simulink model "gm_uz_pmsm_model_9ph_21b_all_double_vnl"  (R2021b)
settings: Solver=FixedStepDiscrete  StartTime=0.0  StopTime=0.8  RelTol=1e-3
PreLoadFcn:
  | uz_pmsm_model_9ph_init_parameter
undefined symbols (not defined in the file or in its folder): a, b, c, friction_coefficient, inertia, k_i_d, k_i_q, k_p_d, k_p_q, Kpd, L_d, L_o1, L_o2, L_q, L_x1, L_x2, L_y1, L_y2, L_zero, polepair, psi_pm, R_1, static_friction_torque, Tnd, ts
libraries: hdlmdlgenlib x139, hdlsllib x90, dspsigops x21, simulink x17, slpidlib x2, spsAlphaBetaZerotodq0Lib x1, pid_lib x1, spsdq0toAlphaBetaZeroLib x1
(part 5 of 5)

== system gm_uz_pmsm_model_9ph_21b_all_double_vnl/uz_pmsm_model_9ph/dq_model_9ph/Data Type Conversion7 ==
  In1 : Inport
  Data Type Conversion7 : DataTypeConversion  OutDataTypeStr=double  RndMeth=Nearest  SampleTime=1e-08
  Data Type Conversion7_pd1 : Delay  DelayLength=3
  Out1 : Outport
  wires:
  Data Type Conversion7_pd1/1 -> Out1/1
  Data Type Conversion7/1 -> Data Type Conversion7_pd1/1
  In1/1 -> Data Type Conversion7/1

== system gm_uz_pmsm_model_9ph_21b_all_double_vnl/uz_pmsm_model_9ph/dq_model_9ph/Data Type Conversion71 ==
  In1 : Inport
  Data Type Conversion71 : DataTypeConversion  OutDataTypeStr=double  RndMeth=Nearest  SampleTime=1e-08
  Data Type Conversion71_pd1 : Delay  DelayLength=3
  Out1 : Outport
  wires:
  Data Type Conversion71_pd1/1 -> Out1/1
  Data Type Conversion71/1 -> Data Type Conversion71_pd1/1
  In1/1 -> Data Type Conversion71/1

== system gm_uz_pmsm_model_9ph_21b_all_double_vnl/uz_pmsm_model_9ph/dq_model_9ph/Data Type Conversion8 ==
  In1 : Inport
  Data Type Conversion8 : DataTypeConversion  OutDataTypeStr=double  RndMeth=Nearest  SampleTime=1e-08
  Data Type Conversion8_pd1 : Delay  DelayLength=3
  Out1 : Outport
  wires:
  Data Type Conversion8_pd1/1 -> Out1/1
  Data Type Conversion8/1 -> Data Type Conversion8_pd1/1
  In1/1 -> Data Type Conversion8/1

== system gm_uz_pmsm_model_9ph_21b_all_double_vnl/uz_pmsm_model_9ph/dq_model_9ph/Data Type Conversion9 ==
  In1 : Inport
  Data Type Conversion9 : DataTypeConversion  OutDataTypeStr=double  RndMeth=Nearest  SampleTime=1e-08
  Data Type Conversion9_pd1 : Delay  DelayLength=3
  Out1 : Outport
  wires:
  Data Type Conversion9_pd1/1 -> Out1/1
  Data Type Conversion9/1 -> Data Type Conversion9_pd1/1
  In1/1 -> Data Type Conversion9/1

== system gm_uz_pmsm_model_9ph_21b_all_double_vnl/uz_pmsm_model_9ph/dq_model_9ph/Divide ==
  In1 : Inport
  In2 : Inport  Port=2
  Divide : Product  Inputs=**  OutDataTypeStr=double  SampleTime=1e-08
  Divide_pd1 : Delay  DelayLength=6
  Out1 : Outport
  wires:
  Divide_pd1/1 -> Out1/1
  Divide/1 -> Divide_pd1/1
  In2/1 -> Divide/2
  In1/1 -> Divide/1

== system gm_uz_pmsm_model_9ph_21b_all_double_vnl/uz_pmsm_model_9ph/dq_model_9ph/Divide1 ==
  In1 : Inport
  In2 : Inport  Port=2
  Divide1 : Product  Inputs=**  OutDataTypeStr=double  SampleTime=1e-08
  Divide1_pd1 : Delay  DelayLength=6
  Out1 : Outport
  wires:
  Divide1_pd1/1 -> Out1/1
  Divide1/1 -> Divide1_pd1/1
  In2/1 -> Divide1/2
  In1/1 -> Divide1/1

== system gm_uz_pmsm_model_9ph_21b_all_double_vnl/uz_pmsm_model_9ph/dq_model_9ph/Divide10 ==
  In1 : Inport
  In2 : Inport  Port=2
  Divide10 : Product  Inputs=**  OutDataTypeStr=double  SampleTime=1e-08
  Divide10_pd1 : Delay  DelayLength=6
  Out1 : Outport
  wires:
  Divide10_pd1/1 -> Out1/1
  Divide10/1 -> Divide10_pd1/1
  In2/1 -> Divide10/2
  In1/1 -> Divide10/1

== system gm_uz_pmsm_model_9ph_21b_all_double_vnl/uz_pmsm_model_9ph/dq_model_9ph/Divide11 ==
  In1 : Inport
  In2 : Inport  Port=2
  Divide11 : Product  Inputs=**  OutDataTypeStr=double  SampleTime=1e-08
  Divide11_pd1 : Delay  DelayLength=6
  Out1 : Outport
  wires:
  Divide11_pd1/1 -> Out1/1
  Divide11/1 -> Divide11_pd1/1
  In2/1 -> Divide11/2
  In1/1 -> Divide11/1

== system gm_uz_pmsm_model_9ph_21b_all_double_vnl/uz_pmsm_model_9ph/dq_model_9ph/Divide12 ==
  In1 : Inport
  In2 : Inport  Port=2
  Divide12 : Product  Inputs=**  OutDataTypeStr=double  SampleTime=1e-08
  Divide12_pd1 : Delay  DelayLength=6
  Out1 : Outport
  wires:
  Divide12_pd1/1 -> Out1/1
  Divide12/1 -> Divide12_pd1/1
  In2/1 -> Divide12/2
  In1/1 -> Divide12/1

== system gm_uz_pmsm_model_9ph_21b_all_double_vnl/uz_pmsm_model_9ph/dq_model_9ph/Divide13 ==
  In1 : Inport
  In2 : Inport  Port=2
  Divide13 : Product  Inputs=**  OutDataTypeStr=double  SampleTime=1e-08
  Divide13_pd1 : Delay  DelayLength=6
  Out1 : Outport
  wires:
  Divide13_pd1/1 -> Out1/1
  Divide13/1 -> Divide13_pd1/1
  In2/1 -> Divide13/2
  In1/1 -> Divide13/1

== system gm_uz_pmsm_model_9ph_21b_all_double_vnl/uz_pmsm_model_9ph/dq_model_9ph/Divide2 ==
  In1 : Inport
  In2 : Inport  Port=2
  Divide2 : Product  Inputs=**  OutDataTypeStr=double  SampleTime=1e-08
  Divide2_pd1 : Delay  DelayLength=6
  Out1 : Outport
  wires:
  Divide2_pd1/1 -> Out1/1
  Divide2/1 -> Divide2_pd1/1
  In2/1 -> Divide2/2
  In1/1 -> Divide2/1

== system gm_uz_pmsm_model_9ph_21b_all_double_vnl/uz_pmsm_model_9ph/dq_model_9ph/Divide3 ==
  In1 : Inport
  In2 : Inport  Port=2
  Divide3 : Product  Inputs=**  OutDataTypeStr=double  SampleTime=1e-08
  Divide3_pd1 : Delay  DelayLength=6
  Out1 : Outport
  wires:
  Divide3_pd1/1 -> Out1/1
  Divide3/1 -> Divide3_pd1/1
  In2/1 -> Divide3/2
  In1/1 -> Divide3/1

== system gm_uz_pmsm_model_9ph_21b_all_double_vnl/uz_pmsm_model_9ph/dq_model_9ph/Divide4 ==
  In1 : Inport
  In2 : Inport  Port=2
  Divide4 : Product  Inputs=**  OutDataTypeStr=double  SampleTime=1e-08
  Divide4_pd1 : Delay  DelayLength=6
  Out1 : Outport
  wires:
  Divide4_pd1/1 -> Out1/1
  Divide4/1 -> Divide4_pd1/1
  In2/1 -> Divide4/2
  In1/1 -> Divide4/1

== system gm_uz_pmsm_model_9ph_21b_all_double_vnl/uz_pmsm_model_9ph/dq_model_9ph/Divide5 ==
  In1 : Inport
  In2 : Inport  Port=2
  Divide5 : Product  Inputs=**  OutDataTypeStr=double  SampleTime=1e-08
  Divide5_pd1 : Delay  DelayLength=6
  Out1 : Outport
  wires:
  Divide5_pd1/1 -> Out1/1
  Divide5/1 -> Divide5_pd1/1
  In2/1 -> Divide5/2
  In1/1 -> Divide5/1

== system gm_uz_pmsm_model_9ph_21b_all_double_vnl/uz_pmsm_model_9ph/dq_model_9ph/Divide6 ==
  In1 : Inport
  In2 : Inport  Port=2
  Divide6 : Product  Inputs=**  OutDataTypeStr=double  SampleTime=1e-08
  Divide6_pd1 : Delay  DelayLength=6
  Out1 : Outport
  wires:
  Divide6_pd1/1 -> Out1/1
  Divide6/1 -> Divide6_pd1/1
  In2/1 -> Divide6/2
  In1/1 -> Divide6/1

== system gm_uz_pmsm_model_9ph_21b_all_double_vnl/uz_pmsm_model_9ph/dq_model_9ph/Divide7 ==
  In1 : Inport
  In2 : Inport  Port=2
  Divide7 : Product  Inputs=**  OutDataTypeStr=double  SampleTime=1e-08
  Divide7_pd1 : Delay  DelayLength=6
  Out1 : Outport
  wires:
  Divide7_pd1/1 -> Out1/1
  Divide7/1 -> Divide7_pd1/1
  In2/1 -> Divide7/2
  In1/1 -> Divide7/1

== system gm_uz_pmsm_model_9ph_21b_all_double_vnl/uz_pmsm_model_9ph/dq_model_9ph/Divide8 ==
  In1 : Inport
  In2 : Inport  Port=2
  Divide8 : Product  Inputs=**  OutDataTypeStr=double  SampleTime=1e-08
  Divide8_pd1 : Delay  DelayLength=6
  Out1 : Outport
  wires:
  Divide8_pd1/1 -> Out1/1
  Divide8/1 -> Divide8_pd1/1
  In2/1 -> Divide8/2
  In1/1 -> Divide8/1

== system gm_uz_pmsm_model_9ph_21b_all_double_vnl/uz_pmsm_model_9ph/dq_model_9ph/Divide9 ==
  In1 : Inport
  In2 : Inport  Port=2
  Divide9 : Product  Inputs=**  OutDataTypeStr=double  SampleTime=1e-08
  Divide9_pd1 : Delay  DelayLength=6
  Out1 : Outport
  wires:
  Divide9_pd1/1 -> Out1/1
  Divide9/1 -> Divide9_pd1/1
  In2/1 -> Divide9/2
  In1/1 -> Divide9/1

== system gm_uz_pmsm_model_9ph_21b_all_double_vnl/uz_pmsm_model_9ph/dq_model_9ph/Factor ==
  In1 : Inport
  In2 : Inport  Port=2
  Factor : Product  Inputs=**  OutDataTypeStr=double  SampleTime=1e-08
  Factor_pd1 : Delay  DelayLength=6
  Out1 : Outport
  wires:
  Factor_pd1/1 -> Out1/1
  Factor/1 -> Factor_pd1/1
  In2/1 -> Factor/2
  In1/1 -> Factor/1

== system gm_uz_pmsm_model_9ph_21b_all_double_vnl/uz_pmsm_model_9ph/dq_model_9ph/Gain ==
  In1 : Inport
  In2 : Inport  Port=2
  Gain : Product  Inputs=**  OutDataTypeStr=double  SampleTime=1e-08
  Gain_pd1 : Delay  DelayLength=6
  Out1 : Outport
  wires:
  Gain_pd1/1 -> Out1/1
  Gain/1 -> Gain_pd1/1
  In2/1 -> Gain/2
  In1/1 -> Gain/1

== system gm_uz_pmsm_model_9ph_21b_all_double_vnl/uz_pmsm_model_9ph/dq_model_9ph/Gain1 ==
  In1 : Inport
  In2 : Inport  Port=2
  Gain1 : Product  Inputs=**  OutDataTypeStr=double  SampleTime=1e-08
  Gain1_pd1 : Delay  DelayLength=6
  Out1 : Outport
  wires:
  Gain1_pd1/1 -> Out1/1
  Gain1/1 -> Gain1_pd1/1
  In2/1 -> Gain1/2
  In1/1 -> Gain1/1

== system gm_uz_pmsm_model_9ph_21b_all_double_vnl/uz_pmsm_model_9ph/dq_model_9ph/Gain10 ==
  In1 : Inport
  In2 : Inport  Port=2
  Gain10 : Product  Inputs=**  OutDataTypeStr=double  SampleTime=1e-08
  Gain10_pd1 : Delay  DelayLength=6
  Out1 : Outport
  wires:
  Gain10_pd1/1 -> Out1/1
  Gain10/1 -> Gain10_pd1/1
  In2/1 -> Gain10/2
  In1/1 -> Gain10/1

== system gm_uz_pmsm_model_9ph_21b_all_double_vnl/uz_pmsm_model_9ph/dq_model_9ph/Gain2 ==
  In1 : Inport
  In2 : Inport  Port=2
  Gain2 : Product  Inputs=**  OutDataTypeStr=double  SampleTime=1e-08
  Gain2_pd1 : Delay  DelayLength=6
  Out1 : Outport
  wires:
  Gain2_pd1/1 -> Out1/1
  Gain2/1 -> Gain2_pd1/1
  In2/1 -> Gain2/2
  In1/1 -> Gain2/1

== system gm_uz_pmsm_model_9ph_21b_all_double_vnl/uz_pmsm_model_9ph/dq_model_9ph/Gain3 ==
  In1 : Inport
  In2 : Inport  Port=2
  Gain3 : Product  Inputs=**  OutDataTypeStr=double  SampleTime=1e-08
  Gain3_pd1 : Delay  DelayLength=6
  Out1 : Outport
  wires:
  Gain3_pd1/1 -> Out1/1
  Gain3/1 -> Gain3_pd1/1
  In2/1 -> Gain3/2
  In1/1 -> Gain3/1

== system gm_uz_pmsm_model_9ph_21b_all_double_vnl/uz_pmsm_model_9ph/dq_model_9ph/Gain4 ==
  In1 : Inport
  In2 : Inport  Port=2
  Gain4 : Product  Inputs=**  OutDataTypeStr=double  SampleTime=1e-08
  Gain4_pd1 : Delay  DelayLength=6
  Out1 : Outport
  wires:
  Gain4_pd1/1 -> Out1/1
  Gain4/1 -> Gain4_pd1/1
  In2/1 -> Gain4/2
  In1/1 -> Gain4/1

== system gm_uz_pmsm_model_9ph_21b_all_double_vnl/uz_pmsm_model_9ph/dq_model_9ph/Gain5 ==
  In1 : Inport
  In2 : Inport  Port=2
  Gain5 : Product  Inputs=**  OutDataTypeStr=double  SampleTime=1e-08
  Gain5_pd1 : Delay  DelayLength=6
  Out1 : Outport
  wires:
  Gain5_pd1/1 -> Out1/1
  Gain5/1 -> Gain5_pd1/1
  In2/1 -> Gain5/2
  In1/1 -> Gain5/1

== system gm_uz_pmsm_model_9ph_21b_all_double_vnl/uz_pmsm_model_9ph/dq_model_9ph/Gain6 ==
  In1 : Inport
  In2 : Inport  Port=2
  Gain6 : Product  Inputs=**  OutDataTypeStr=double  SampleTime=1e-08
  Gain6_pd1 : Delay  DelayLength=6
  Out1 : Outport
  wires:
  Gain6_pd1/1 -> Out1/1
  Gain6/1 -> Gain6_pd1/1
  In2/1 -> Gain6/2
  In1/1 -> Gain6/1

== system gm_uz_pmsm_model_9ph_21b_all_double_vnl/uz_pmsm_model_9ph/dq_model_9ph/Gain7 ==
  In1 : Inport
  In2 : Inport  Port=2
  Gain7 : Product  Inputs=**  OutDataTypeStr=double  SampleTime=1e-08
  Gain7_pd1 : Delay  DelayLength=6
  Out1 : Outport
  wires:
  Gain7_pd1/1 -> Out1/1
  Gain7/1 -> Gain7_pd1/1
  In2/1 -> Gain7/2
  In1/1 -> Gain7/1

== system gm_uz_pmsm_model_9ph_21b_all_double_vnl/uz_pmsm_model_9ph/dq_model_9ph/Gain8 ==
  In1 : Inport
  In2 : Inport  Port=2
  Gain8 : Product  Inputs=**  OutDataTypeStr=double  SampleTime=1e-08
  Gain8_pd1 : Delay  DelayLength=6
  Out1 : Outport
  wires:
  Gain8_pd1/1 -> Out1/1
  Gain8/1 -> Gain8_pd1/1
  In2/1 -> Gain8/2
  In1/1 -> Gain8/1

== system gm_uz_pmsm_model_9ph_21b_all_double_vnl/uz_pmsm_model_9ph/dq_model_9ph/Gain9 ==
  In1 : Inport
  In2 : Inport  Port=2
  Gain9 : Product  Inputs=**  OutDataTypeStr=double  SampleTime=1e-08
  Gain9_pd1 : Delay  DelayLength=6
  Out1 : Outport
  wires:
  Gain9_pd1/1 -> Out1/1
  Gain9/1 -> Gain9_pd1/1
  In2/1 -> Gain9/2
  In1/1 -> Gain9/1

== system gm_uz_pmsm_model_9ph_21b_all_double_vnl/uz_pmsm_model_9ph/dq_model_9ph/Product ==
  In1 : Inport
  In2 : Inport  Port=2
  Product : Product  Inputs=**  OutDataTypeStr=double  SampleTime=1e-08
  Product_pd1 : Delay  DelayLength=6
  Out1 : Outport
  wires:
  Product_pd1/1 -> Out1/1
  Product/1 -> Product_pd1/1
  In2/1 -> Product/2
  In1/1 -> Product/1

== system gm_uz_pmsm_model_9ph_21b_all_double_vnl/uz_pmsm_model_9ph/dq_model_9ph/Product1 ==
  In1 : Inport
  In2 : Inport  Port=2
  Product1 : Product  Inputs=**  OutDataTypeStr=double  SampleTime=1e-08
  Product1_pd1 : Delay  DelayLength=6
  Out1 : Outport
  wires:
  Product1_pd1/1 -> Out1/1
  Product1/1 -> Product1_pd1/1
  In2/1 -> Product1/2
  In1/1 -> Product1/1

== system gm_uz_pmsm_model_9ph_21b_all_double_vnl/uz_pmsm_model_9ph/dq_model_9ph/Product10 ==
  In1 : Inport
  In2 : Inport  Port=2
  Product10 : Product  Inputs=**  OutDataTypeStr=double  SampleTime=1e-08
  Product10_pd1 : Delay  DelayLength=6
  Out1 : Outport
  wires:
  Product10_pd1/1 -> Out1/1
  Product10/1 -> Product10_pd1/1
  In2/1 -> Product10/2
  In1/1 -> Product10/1

== system gm_uz_pmsm_model_9ph_21b_all_double_vnl/uz_pmsm_model_9ph/dq_model_9ph/Product11 ==
  In1 : Inport
  In2 : Inport  Port=2
  Product11 : Product  Inputs=**  OutDataTypeStr=double  SampleTime=1e-08
  Product11_pd1 : Delay  DelayLength=6
  Out1 : Outport
  wires:
  Product11_pd1/1 -> Out1/1
  Product11/1 -> Product11_pd1/1
  In2/1 -> Product11/2
  In1/1 -> Product11/1

== system gm_uz_pmsm_model_9ph_21b_all_double_vnl/uz_pmsm_model_9ph/dq_model_9ph/Product2 ==
  In1 : Inport
  In2 : Inport  Port=2
  Product2 : Product  Inputs=**  OutDataTypeStr=double  SampleTime=1e-08
  Product2_pd1 : Delay  DelayLength=6
  Out1 : Outport
  wires:
  Product2_pd1/1 -> Out1/1
  Product2/1 -> Product2_pd1/1
  In2/1 -> Product2/2
  In1/1 -> Product2/1

== system gm_uz_pmsm_model_9ph_21b_all_double_vnl/uz_pmsm_model_9ph/dq_model_9ph/Product3 ==
  In1 : Inport
  In2 : Inport  Port=2
  Product3 : Product  Inputs=**  OutDataTypeStr=double  SampleTime=1e-08
  Product3_pd1 : Delay  DelayLength=6
  Out1 : Outport
  wires:
  Product3_pd1/1 -> Out1/1
  Product3/1 -> Product3_pd1/1
  In2/1 -> Product3/2
  In1/1 -> Product3/1

== system gm_uz_pmsm_model_9ph_21b_all_double_vnl/uz_pmsm_model_9ph/dq_model_9ph/Product4 ==
  In1 : Inport
  In2 : Inport  Port=2
  Product4 : Product  Inputs=**  OutDataTypeStr=double  SampleTime=1e-08
  Product4_pd1 : Delay  DelayLength=6
  Out1 : Outport
  wires:
  Product4_pd1/1 -> Out1/1
  Product4/1 -> Product4_pd1/1
  In2/1 -> Product4/2
  In1/1 -> Product4/1

== system gm_uz_pmsm_model_9ph_21b_all_double_vnl/uz_pmsm_model_9ph/dq_model_9ph/Product5 ==
  In1 : Inport
  In2 : Inport  Port=2
  Product5 : Product  Inputs=**  OutDataTypeStr=double  SampleTime=1e-08
  Product5_pd1 : Delay  DelayLength=6
  Out1 : Outport
  wires:
  Product5_pd1/1 -> Out1/1
  Product5/1 -> Product5_pd1/1
  In2/1 -> Product5/2
  In1/1 -> Product5/1

== system gm_uz_pmsm_model_9ph_21b_all_double_vnl/uz_pmsm_model_9ph/dq_model_9ph/Product6 ==
  In1 : Inport
  In2 : Inport  Port=2
  Product6 : Product  Inputs=**  OutDataTypeStr=double  SampleTime=1e-08
  Product6_pd1 : Delay  DelayLength=6
  Out1 : Outport
  wires:
  Product6_pd1/1 -> Out1/1
  Product6/1 -> Product6_pd1/1
  In2/1 -> Product6/2
  In1/1 -> Product6/1

== system gm_uz_pmsm_model_9ph_21b_all_double_vnl/uz_pmsm_model_9ph/dq_model_9ph/Product7 ==
  In1 : Inport
  In2 : Inport  Port=2
  Product7 : Product  Inputs=**  OutDataTypeStr=double  SampleTime=1e-08
  Product7_pd1 : Delay  DelayLength=6
  Out1 : Outport
  wires:
  Product7_pd1/1 -> Out1/1
  Product7/1 -> Product7_pd1/1
  In2/1 -> Product7/2
  In1/1 -> Product7/1

== system gm_uz_pmsm_model_9ph_21b_all_double_vnl/uz_pmsm_model_9ph/dq_model_9ph/Product8 ==
  In1 : Inport
  In2 : Inport  Port=2
  Product8 : Product  Inputs=**  OutDataTypeStr=double  SampleTime=1e-08
  Product8_pd1 : Delay  DelayLength=6
  Out1 : Outport
  wires:
  Product8_pd1/1 -> Out1/1
  Product8/1 -> Product8_pd1/1
  In2/1 -> Product8/2
  In1/1 -> Product8/1

== system gm_uz_pmsm_model_9ph_21b_all_double_vnl/uz_pmsm_model_9ph/dq_model_9ph/Product9 ==
  In1 : Inport
  In2 : Inport  Port=2
  Product9 : Product  Inputs=**  OutDataTypeStr=double  SampleTime=1e-08
  Product9_pd1 : Delay  DelayLength=6
  Out1 : Outport
  wires:
  Product9_pd1/1 -> Out1/1
  Product9/1 -> Product9_pd1/1
  In2/1 -> Product9/2
  In1/1 -> Product9/1

== system gm_uz_pmsm_model_9ph_21b_all_double_vnl/uz_pmsm_model_9ph/dq_model_9ph/Sum ==
  In1 : Inport
  In2 : Inport  Port=2
  Sum : Sum  OutDataTypeStr=double  SampleTime=1e-08
  Sum_pd1 : Delay  DelayLength=6
  Out1 : Outport
  wires:
  Sum_pd1/1 -> Out1/1
  Sum/1 -> Sum_pd1/1
  In2/1 -> Sum/2
  In1/1 -> Sum/1

== system gm_uz_pmsm_model_9ph_21b_all_double_vnl/uz_pmsm_model_9ph/dq_model_9ph/Sum1 ==
  In1 : Inport
  In2 : Inport  Port=2
  Sum1 : Sum  Inputs=+-  OutDataTypeStr=double  SampleTime=1e-08
  Sum1_pd1 : Delay  DelayLength=6
  Out1 : Outport
  wires:
  Sum1_pd1/1 -> Out1/1
  Sum1/1 -> Sum1_pd1/1
  In2/1 -> Sum1/2
  In1/1 -> Sum1/1

== system gm_uz_pmsm_model_9ph_21b_all_double_vnl/uz_pmsm_model_9ph/dq_model_9ph/Sum11 ==
  In1 : Inport
  In2 : Inport  Port=2
  Sum11 : Sum  OutDataTypeStr=double  SampleTime=1e-08
  Sum11_pd1 : Delay  DelayLength=6
  Out1 : Outport
  wires:
  Sum11_pd1/1 -> Out1/1
  Sum11/1 -> Sum11_pd1/1
  In2/1 -> Sum11/2
  In1/1 -> Sum11/1

== system gm_uz_pmsm_model_9ph_21b_all_double_vnl/uz_pmsm_model_9ph/dq_model_9ph/Sum1_stage2 ==
  In1 : Inport
  In2 : Inport  Port=2
  Sum1_stage2 : Sum  Inputs=+-  OutDataTypeStr=double  SampleTime=1e-08
  Sum1_stage2_pd1 : Delay  DelayLength=6
  Out1 : Outport
  wires:
  Sum1_stage2_pd1/1 -> Out1/1
  Sum1_stage2/1 -> Sum1_stage2_pd1/1
  In2/1 -> Sum1_stage2/2
  In1/1 -> Sum1_stage2/1

== system gm_uz_pmsm_model_9ph_21b_all_double_vnl/uz_pmsm_model_9ph/dq_model_9ph/Sum1_stage3 ==
  In1 : Inport
  In2 : Inport  Port=2
  Sum1_stage3 : Sum  Inputs=+-  OutDataTypeStr=double  SampleTime=1e-08
  Sum1_stage3_pd1 : Delay  DelayLength=6
  Out1 : Outport
  wires:
  Sum1_stage3_pd1/1 -> Out1/1
  Sum1_stage3/1 -> Sum1_stage3_pd1/1
  In2/1 -> Sum1_stage3/2
  In1/1 -> Sum1_stage3/1

== system gm_uz_pmsm_model_9ph_21b_all_double_vnl/uz_pmsm_model_9ph/dq_model_9ph/Sum2 ==
  In1 : Inport
  In2 : Inport  Port=2
  Sum2 : Sum  OutDataTypeStr=double  SampleTime=1e-08
  Sum2_pd1 : Delay  DelayLength=6
  Out1 : Outport
  wires:
  Sum2_pd1/1 -> Out1/1
  Sum2/1 -> Sum2_pd1/1
  In2/1 -> Sum2/2
  In1/1 -> Sum2/1

== system gm_uz_pmsm_model_9ph_21b_all_double_vnl/uz_pmsm_model_9ph/dq_model_9ph/Sum21 ==
  In1 : Inport
  In2 : Inport  Port=2
  Sum21 : Sum  Inputs=+-  OutDataTypeStr=double  SampleTime=1e-08
  Sum21_pd1 : Delay  DelayLength=6
  Out1 : Outport
  wires:
  Sum21_pd1/1 -> Out1/1
  Sum21/1 -> Sum21_pd1/1
  In2/1 -> Sum21/2
  In1/1 -> Sum21/1

== system gm_uz_pmsm_model_9ph_21b_all_double_vnl/uz_pmsm_model_9ph/dq_model_9ph/Sum3 ==
  In1 : Inport
  In2 : Inport  Port=2
  Sum3 : Sum  OutDataTypeStr=double  SampleTime=1e-08
  Sum3_pd1 : Delay  DelayLength=6
  Out1 : Outport
  wires:
  Sum3_pd1/1 -> Out1/1
  Sum3/1 -> Sum3_pd1/1
  In2/1 -> Sum3/2
  In1/1 -> Sum3/1

== system gm_uz_pmsm_model_9ph_21b_all_double_vnl/uz_pmsm_model_9ph/dq_model_9ph/Sum31 ==
  In1 : Inport
  In2 : Inport  Port=2
  Sum31 : Sum  OutDataTypeStr=double  SampleTime=1e-08
  Sum31_pd1 : Delay  DelayLength=6
  Out1 : Outport
  wires:
  Sum31_pd1/1 -> Out1/1
  Sum31/1 -> Sum31_pd1/1
  In2/1 -> Sum31/2
  In1/1 -> Sum31/1

== system gm_uz_pmsm_model_9ph_21b_all_double_vnl/uz_pmsm_model_9ph/dq_model_9ph/Sum310 ==
  In1 : Inport
  In2 : Inport  Port=2
  Sum310 : Sum  OutDataTypeStr=double  SampleTime=1e-08
  Sum310_pd1 : Delay  DelayLength=6
  Out1 : Outport
  wires:
  Sum310_pd1/1 -> Out1/1
  Sum310/1 -> Sum310_pd1/1
  In2/1 -> Sum310/2
  In1/1 -> Sum310/1

== system gm_uz_pmsm_model_9ph_21b_all_double_vnl/uz_pmsm_model_9ph/dq_model_9ph/Sum32 ==
  In1 : Inport
  In2 : Inport  Port=2
  Sum32 : Sum  OutDataTypeStr=double  SampleTime=1e-08
  Sum32_pd1 : Delay  DelayLength=6
  Out1 : Outport
  wires:
  Sum32_pd1/1 -> Out1/1
  Sum32/1 -> Sum32_pd1/1
  In2/1 -> Sum32/2
  In1/1 -> Sum32/1

== system gm_uz_pmsm_model_9ph_21b_all_double_vnl/uz_pmsm_model_9ph/dq_model_9ph/Sum33 ==
  In1 : Inport
  In2 : Inport  Port=2
  Sum33 : Sum  OutDataTypeStr=double  SampleTime=1e-08
  Sum33_pd1 : Delay  DelayLength=6
  Out1 : Outport
  wires:
  Sum33_pd1/1 -> Out1/1
  Sum33/1 -> Sum33_pd1/1
  In2/1 -> Sum33/2
  In1/1 -> Sum33/1

== system gm_uz_pmsm_model_9ph_21b_all_double_vnl/uz_pmsm_model_9ph/dq_model_9ph/Sum34 ==
  In1 : Inport
  In2 : Inport  Port=2
  Sum34 : Sum  OutDataTypeStr=double  SampleTime=1e-08
  Sum34_pd1 : Delay  DelayLength=6
  Out1 : Outport
  wires:
  Sum34_pd1/1 -> Out1/1
  Sum34/1 -> Sum34_pd1/1
  In2/1 -> Sum34/2
  In1/1 -> Sum34/1

== system gm_uz_pmsm_model_9ph_21b_all_double_vnl/uz_pmsm_model_9ph/dq_model_9ph/Sum35 ==
  In1 : Inport
  In2 : Inport  Port=2
  Sum35 : Sum  OutDataTypeStr=double  SampleTime=1e-08
  Sum35_pd1 : Delay  DelayLength=6
  Out1 : Outport
  wires:
  Sum35_pd1/1 -> Out1/1
  Sum35/1 -> Sum35_pd1/1
  In2/1 -> Sum35/2
  In1/1 -> Sum35/1

== system gm_uz_pmsm_model_9ph_21b_all_double_vnl/uz_pmsm_model_9ph/dq_model_9ph/Sum36 ==
  In1 : Inport
  In2 : Inport  Port=2
  Sum36 : Sum  OutDataTypeStr=double  SampleTime=1e-08
  Sum36_pd1 : Delay  DelayLength=6
  Out1 : Outport
  wires:
  Sum36_pd1/1 -> Out1/1
  Sum36/1 -> Sum36_pd1/1
  In2/1 -> Sum36/2
  In1/1 -> Sum36/1

== system gm_uz_pmsm_model_9ph_21b_all_double_vnl/uz_pmsm_model_9ph/dq_model_9ph/Sum37 ==
  In1 : Inport
  In2 : Inport  Port=2
  Sum37 : Sum  OutDataTypeStr=double  SampleTime=1e-08
  Sum37_pd1 : Delay  DelayLength=6
  Out1 : Outport
  wires:
  Sum37_pd1/1 -> Out1/1
  Sum37/1 -> Sum37_pd1/1
  In2/1 -> Sum37/2
  In1/1 -> Sum37/1

== system gm_uz_pmsm_model_9ph_21b_all_double_vnl/uz_pmsm_model_9ph/dq_model_9ph/Sum38 ==
  In1 : Inport
  In2 : Inport  Port=2
  Sum38 : Sum  Inputs=+-  OutDataTypeStr=double  SampleTime=1e-08
  Sum38_pd1 : Delay  DelayLength=6
  Out1 : Outport
  wires:
  Sum38_pd1/1 -> Out1/1
  Sum38/1 -> Sum38_pd1/1
  In2/1 -> Sum38/2
  In1/1 -> Sum38/1

== system gm_uz_pmsm_model_9ph_21b_all_double_vnl/uz_pmsm_model_9ph/dq_model_9ph/Sum39 ==
  In1 : Inport
  In2 : Inport  Port=2
  Sum39 : Sum  OutDataTypeStr=double  SampleTime=1e-08
  Sum39_pd1 : Delay  DelayLength=6
  Out1 : Outport
  wires:
  Sum39_pd1/1 -> Out1/1
  Sum39/1 -> Sum39_pd1/1
  In2/1 -> Sum39/2
  In1/1 -> Sum39/1

== system gm_uz_pmsm_model_9ph_21b_all_double_vnl/uz_pmsm_model_9ph/dq_model_9ph/Sum_stage2 ==
  In1 : Inport
  In2 : Inport  Port=2
  Sum_stage2 : Sum  Inputs=+-  OutDataTypeStr=double  SampleTime=1e-08
  Sum_stage2_pd1 : Delay  DelayLength=6
  Out1 : Outport
  wires:
  Sum_stage2_pd1/1 -> Out1/1
  Sum_stage2/1 -> Sum_stage2_pd1/1
  In2/1 -> Sum_stage2/2
  In1/1 -> Sum_stage2/1

== system gm_uz_pmsm_model_9ph_21b_all_double_vnl/uz_pmsm_model_9ph/dq_model_9ph/Sum_stage3 ==
  In1 : Inport
  In2 : Inport  Port=2
  Sum_stage3 : Sum  OutDataTypeStr=double  SampleTime=1e-08
  Sum_stage3_pd1 : Delay  DelayLength=6
  Out1 : Outport
  wires:
  Sum_stage3_pd1/1 -> Out1/1
  Sum_stage3/1 -> Sum_stage3_pd1/1
  In2/1 -> Sum_stage3/2
  In1/1 -> Sum_stage3/1

== system gm_uz_pmsm_model_9ph_21b_all_double_vnl/uz_pmsm_model_9ph_vnl/Line-Line to Phase voltage/abc   to   alpha_beta_0 ==
  "a, b, c" : Inport  PortDimensions=3
  Gain2 : Gain  Gain=2/3  ParamDataTypeStr=fixdt(1,18,16)  SaturateOnIntegerOverflow=on  OutDataTypeStr=Inherit: Same as input
  Gain4 : Gain  Gain="[ 1   -0.5   -0.5; 0   0.5*sqrt(3)   -0.5*sqrt(3); 0.5  0.5  0.5 ]"  Multiplication=Matrix(K*u) (u vector)  ParamDataTypeStr=fixdt(1,18,16)  OutDataTypeStr=fixdt(1,25,12)  SaturateOnIntegerOverflow=on
  "alpha, beta, 0 " : Outport
  wires:
  Gain4/1 -> Gain2/1
  "a, b, c"/1 -> Gain4/1
  Gain2/1 -> "alpha, beta, 0 "/1

== system gm_uz_pmsm_model_9ph_21b_all_double_vnl/uz_pmsm_model_9ph_vnl/Line-Line to Phase voltage/alpha_beta_0   to   abc ==
  "alpha, beta, 0  " : Inport  PortDimensions=3
  Gain4 : Gain  Gain="[ 1 0 1; -0.5   0.5*sqrt(3)  1; -0.5 -0.5*sqrt(3) 1 ]"  Multiplication=Matrix(K*u) (u vector)  ParamDataTypeStr=fixdt(1,18,16)  SaturateOnIntegerOverflow=on  OutDataTypeStr=Inherit: Same as input
  "a, b, c" : Outport
  wires:
  "alpha, beta, 0  "/1 -> Gain4/1
  Gain4/1 -> "a, b, c"/1

== system gm_uz_pmsm_model_9ph_21b_all_double_vnl/uz_pmsm_model_9ph_vnl/Line-Line to Phase voltage1/abc   to   alpha_beta_0 ==
  "a, b, c" : Inport  PortDimensions=3
  Gain2 : Gain  Gain=2/3  ParamDataTypeStr=fixdt(1,18,16)  SaturateOnIntegerOverflow=on  OutDataTypeStr=Inherit: Same as input
  Gain4 : Gain  Gain="[ 1   -0.5   -0.5; 0   0.5*sqrt(3)   -0.5*sqrt(3); 0.5  0.5  0.5 ]"  Multiplication=Matrix(K*u) (u vector)  ParamDataTypeStr=fixdt(1,18,16)  OutDataTypeStr=fixdt(1,25,12)  SaturateOnIntegerOverflow=on
  "alpha, beta, 0 " : Outport
  wires:
  Gain2/1 -> "alpha, beta, 0 "/1
  "a, b, c"/1 -> Gain4/1
  Gain4/1 -> Gain2/1

== system gm_uz_pmsm_model_9ph_21b_all_double_vnl/uz_pmsm_model_9ph_vnl/Line-Line to Phase voltage1/alpha_beta_0   to   abc ==
  "alpha, beta, 0  " : Inport  PortDimensions=3
  Gain4 : Gain  Gain="[ 1 0 1; -0.5   0.5*sqrt(3)  1; -0.5 -0.5*sqrt(3) 1 ]"  Multiplication=Matrix(K*u) (u vector)  ParamDataTypeStr=fixdt(1,18,16)  SaturateOnIntegerOverflow=on  OutDataTypeStr=Inherit: Same as input
  "a, b, c" : Outport
  wires:
  Gain4/1 -> "a, b, c"/1
  "alpha, beta, 0  "/1 -> Gain4/1

== system gm_uz_pmsm_model_9ph_21b_all_double_vnl/uz_pmsm_model_9ph_vnl/Line-Line to Phase voltage2/abc   to   alpha_beta_0 ==
  "a, b, c" : Inport  PortDimensions=3
  Gain2 : Gain  Gain=2/3  ParamDataTypeStr=fixdt(1,18,16)  SaturateOnIntegerOverflow=on  OutDataTypeStr=Inherit: Same as input
  Gain4 : Gain  Gain="[ 1   -0.5   -0.5; 0   0.5*sqrt(3)   -0.5*sqrt(3); 0.5  0.5  0.5 ]"  Multiplication=Matrix(K*u) (u vector)  ParamDataTypeStr=fixdt(1,18,16)  OutDataTypeStr=fixdt(1,25,12)  SaturateOnIntegerOverflow=on
  "alpha, beta, 0 " : Outport
  wires:
  Gain4/1 -> Gain2/1
  "a, b, c"/1 -> Gain4/1
  Gain2/1 -> "alpha, beta, 0 "/1

== system gm_uz_pmsm_model_9ph_21b_all_double_vnl/uz_pmsm_model_9ph_vnl/Line-Line to Phase voltage2/alpha_beta_0   to   abc ==
  "alpha, beta, 0  " : Inport  PortDimensions=3
  Gain4 : Gain  Gain="[ 1 0 1; -0.5   0.5*sqrt(3)  1; -0.5 -0.5*sqrt(3) 1 ]"  Multiplication=Matrix(K*u) (u vector)  ParamDataTypeStr=fixdt(1,18,16)  SaturateOnIntegerOverflow=on  OutDataTypeStr=Inherit: Same as input
  "a, b, c" : Outport
  wires:
  "alpha, beta, 0  "/1 -> Gain4/1
  Gain4/1 -> "a, b, c"/1

== system gm_uz_pmsm_model_9ph_21b_all_double_vnl/uz_pmsm_model_9ph_vnl/dq_model_9ph/Wrapped State DTI ==
  note: https://de.mathworks.com/help/releases/R2021a/hdlcoder/ug/troubleshoot-generate-implementation-model-from-simscape-pmsm.html?searchHighlight=troubleshoot-generate-implementation-model-from-simscape-pmsm&s_tid=doc_srchtitle
  Angular Speed : Inport
  polepair : Inport  Port=2
  reset : Inport  Port=3
  Compare To Constant : simulink/Logic and Bit Operations/Compare To Constant  relop=>=  const=single(pi)  OutDataTypeStr=boolean
  Compare To Constant1 : simulink/Logic and Bit Operations/Compare To Constant  relop=<  const=single(-pi)  OutDataTypeStr=boolean
  Constant : Constant  Value=double(2*pi)  SampleTime=-1
  Delay1 : Delay  DelayLength=1  ExternalReset=Level
      settings: InputPortMap=u0,r5
  Gain : Gain  Gain=ts
  Product : Product
  Sum : Sum  Inputs=|++
  Sum1 : Sum  Inputs=|-+
  Sum2 : Sum  Inputs=|++
  Switch : Switch  Criteria=u2 > Threshold
  Switch1 : Switch  Criteria=u2 > Threshold
  Angular Position : Outport
  wires:
  polepair/1 -> Product/2
  Angular Speed/1 -> Product/1
  Product/1 -> Gain/1
  reset/1 -> Delay1/2
  Gain/1 -> Sum/2
  Sum1/1 -> Switch/1
  Sum/1 -> Switch/3, Sum1/2, Compare To Constant/1
  Compare To Constant/1 -> Switch/2
  Switch/1 -> Switch1/3, Compare To Constant1/1, Sum2/2
  Switch1/1 -> Delay1/1  "Angular Position"
  Sum2/1 -> Switch1/1
  Constant/1 -> Sum1/1, Sum2/1
  Delay1/1 -> Angular Position/1, Sum/1
  Compare To Constant1/1 -> Switch1/2

== system gm_uz_pmsm_model_9ph_21b_all_double_vnl/uz_pmsm_model_9ph_vnl/dq_model_9ph/mechanical_system ==
  note: This delay breaks the algebraic loop between mechanical and electrical system.
      | Introduces a delay of 500ns.
  note: load torque negative!!!
  reset : Inport
  M_Mi : Inport  Port=2
  reciprocal_J : Inport  Port=3
  load_torque : Inport  Port=4
  Delay : Delay  DelayLength=1
  Product11 : Product
  Sum1 : Sum  Inputs=|++
  integrator : Subsystem
  omega_mech : Outport
  wires:
  reset/1 -> integrator/2(reset)
  Product11/1 -> integrator/1(in)
  integrator/1(outt) -> omega_mech/1
  Delay/1 -> Sum1/1
  M_Mi/1 -> Delay/1
  load_torque/1 -> Sum1/2
  Sum1/1 -> Product11/2
  reciprocal_J/1 -> Product11/1

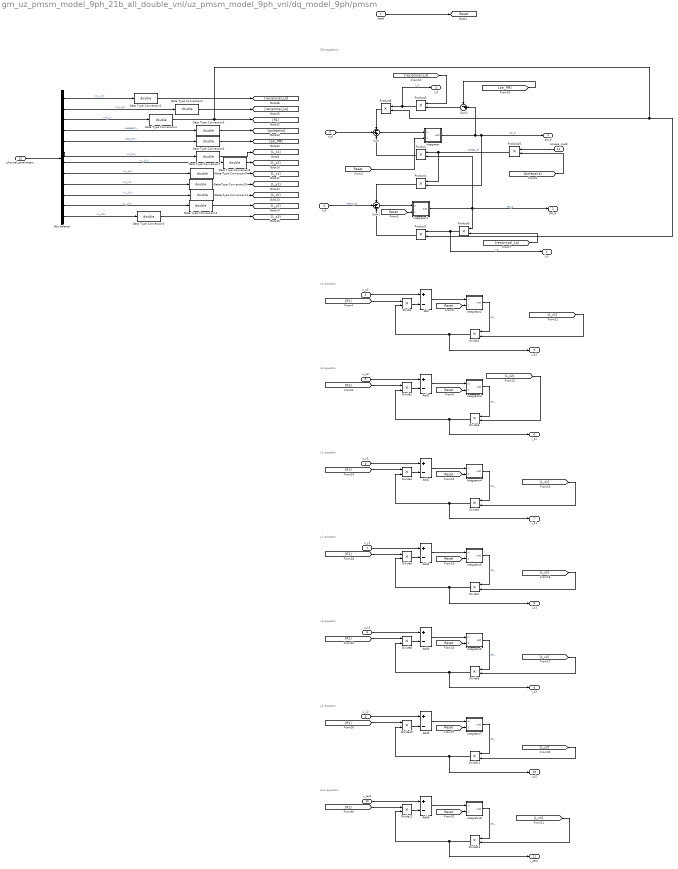
== system gm_uz_pmsm_model_9ph_21b_all_double_vnl/uz_pmsm_model_9ph_vnl/dq_model_9ph/pmsm ==
  note: zero equation
  note: y2 equation
  note: x2 equation
  note: y1 equation
  note: x1 equation
  note: o2 equation
  note: DQ equations
  note: o1 equation
  reset : Inport
  u_d : Inport  Port=2
  u_q : Inport  Port=3
  u_o1 : Inport  Port=4
  u_o2 : Inport  Port=5
  u_x1 : Inport  Port=6
  u_y1 : Inport  Port=7
  u_x2 : Inport  Port=8
  u_y2 : Inport  Port=9
  u_zero : Inport  Port=10
  omega_mech : Inport  Port=11
  physical_parameters : Inport  Port=12
  Add{,1..6} (7 alike) : Sum  Inputs=+-
  Bus Selector : BusSelector  OutputSignals=1_L_d,1_L_q,R_1,polepair,psi_pm,L_z1,L_z2,L_x1,L_y1,L_x2,L_y2,L_z3
  Data Type Conversion{1..12} (12 alike) : DataTypeConversion  OutDataTypeStr=double  RndMeth=Nearest
  Divide{,1..13} (14 alike) : Product  Inputs=**
  Product{,1,5..8,10} (7 alike) : Product
  Sum : Sum  Inputs=-++
  Sum1 : Sum  Inputs=-+-
  Sum2 : Sum  Inputs=-+|
  integrator : Subsystem
  integrator1 : Subsystem
  integrator2 : Subsystem
  integrator3 : Subsystem
  integrator4 : Subsystem
  integrator5 : Subsystem
  integrator6 : Subsystem
  integrator7 : Subsystem
  integrator8 : Subsystem
  psi_d : Outport
  psi_q : Outport  Port=2
  I_d : Outport  Port=3
  I_q : Outport  Port=4
  i_o1 : Outport  Port=5
  i_o2 : Outport  Port=6
  i_x1 : Outport  Port=7
  i_y1 : Outport  Port=8
  i_x2 : Outport  Port=9
  i_y2 : Outport  Port=10
  i_zero : Outport  Port=11
  tag scope: Reset=global
  wires:
  Data Type Conversion12/1 -> [L_y2]
  Data Type Conversion11/1 -> [L_x2]
  Data Type Conversion10/1 -> [L_y1]
  Data Type Conversion9/1 -> [L_x1]
  Data Type Conversion8/1 -> [L_z2]
  Data Type Conversion7/1 -> [L_z1]
  Data Type Conversion6/1 -> [psi_PM]
  Data Type Conversion5/1 -> [polepairs]
  Data Type Conversion4/1 -> Product8/2, Product7/2, [R1]
  Data Type Conversion2/1 -> [reciprocal_Lq]
  Bus Selector/12 -> Data Type Conversion3/1  "<L_z3>"
  Data Type Conversion3/1 -> [L_z3]
  Data Type Conversion1/1 -> [reciprocal_Ld]
  u_d/1 -> Sum/2
  Add6/1 -> integrator8/1(in)
  Add5/1 -> integrator7/1(in)
  Add4/1 -> integrator6/1(in)
  Add3/1 -> integrator5/1(in)
  Add2/1 -> integrator4/1(in)
  Add1/1 -> integrator3/1(in)
  Add/1 -> integrator2/1(in)
  Sum1/1 -> integrator1/1(in)
  Sum/1 -> integrator/1(in)
  [L_z3] -> Divide13/2
  [L_y2] -> Divide11/2
  [L_x2] -> Divide9/2
  [L_y1] -> Divide7/2
  [L_x1] -> Divide5/2
  [polepairs] -> Product10/2
  Bus Selector/9 -> Data Type Conversion10/1  "<L_y1>"
  physical_parameters/1 -> Bus Selector/1
  Bus Selector/10 -> Data Type Conversion11/1  "<L_x2>"
  Bus Selector/3 -> Data Type Conversion4/1  "<R_1>"
  Bus Selector/11 -> Data Type Conversion12/1  "<L_y2>"
  Bus Selector/7 -> Data Type Conversion8/1  "<L_z2>"
  Bus Selector/6 -> Data Type Conversion7/1  "<L_z1>"
  Bus Selector/5 -> Data Type Conversion6/1  "<psi_pm>"
  Bus Selector/2 -> Data Type Conversion2/1  "<1_L_q>"
  Bus Selector/8 -> Data Type Conversion9/1  "<L_x1>"
  Bus Selector/4 -> Data Type Conversion5/1  "<polepair>"
  Bus Selector/1 -> Data Type Conversion1/1  "<1_L_d>"
  integrator8/1(outt) -> Divide13/1  "psi_"
  [R1] -> Divide12/1
  Divide12/1 -> Add6/2
  Divide13/1 -> Divide12/2, i_zero/1
  u_zero/1 -> Add6/1
  [Reset] -> integrator8/2(reset)
  [Reset] -> integrator7/2(reset)
  u_y2/1 -> Add5/1
  Divide11/1 -> Divide10/2, i_y2/1
  Divide10/1 -> Add5/2
  [R1] -> Divide10/1
  integrator7/1(outt) -> Divide11/1  "psi_"
  integrator6/1(outt) -> Divide9/1  "psi_"
  [R1] -> Divide8/1
  Divide8/1 -> Add4/2
  Divide9/1 -> Divide8/2, i_x2/1
  u_x2/1 -> Add4/1
  [Reset] -> integrator6/2(reset)
  [Reset] -> integrator5/2(reset)
  u_y1/1 -> Add3/1
  Divide7/1 -> Divide6/2, i_y1/1
  Divide6/1 -> Add3/2
  [R1] -> Divide6/1
  integrator5/1(outt) -> Divide7/1  "psi_"
  integrator4/1(outt) -> Divide5/1  "psi_"
  [R1] -> Divide4/1
  Divide4/1 -> Add2/2
  Divide5/1 -> Divide4/2, i_x1/1
  u_x1/1 -> Add2/1
  [Reset] -> integrator4/2(reset)
  [Reset] -> integrator3/2(reset)
  [L_z2] -> Divide3/2
  u_o2/1 -> Add1/1
  Divide3/1 -> Divide2/2, i_o2/1
  Divide2/1 -> Add1/2
  [R1] -> Divide2/1
  integrator3/1(outt) -> Divide3/1  "psi_"
  integrator2/1(outt) -> Divide1/1  "psi_"
  [R1] -> Divide/1
  Divide/1 -> Add/2
  Divide1/1 -> Divide/2, i_o1/1
  u_o1/1 -> Add/1
  [L_z1] -> Divide1/2
  [Reset] -> integrator2/2(reset)
  [Reset] -> integrator1/2(reset)
  [Reset] -> integrator/2(reset)
  reset/1 -> [Reset]
  Product7/1 -> Sum1/3
  [reciprocal_Lq] -> Product6/2
  Product8/1 -> Sum/1
  Sum2/1 -> Product5/2
  integrator/1(outt) -> Product1/2, psi_d/1, Sum2/2  "psi_d"
  Product10/1 -> Product/1, Product1/1  "omega_el"
  Product6/1 -> Product7/1, I_q/1  "I_q"
  [psi_PM] -> Sum2/1
  Product1/1 -> Sum1/1
  integrator1/1(outt) -> Product6/1, Product/2, psi_q/1  "psi_q"
  [reciprocal_Ld] -> Product5/1
  Product5/1 -> Product8/1, I_d/1  "I_d"
  Product/1 -> Sum/3
  u_q/1 -> Sum1/2  "intern_uq"
  omega_mech/1 -> Product10/1

== system gm_uz_pmsm_model_9ph_21b_all_double_vnl/uz_pmsm_model_9ph_vnl/dq_model_9ph/torque_calculation ==
  I_d : Inport
  I_q : Inport  Port=2
  psi_d : Inport  Port=3
  psi_q : Inport  Port=4
  polepairs : Inport  Port=5
  Factor : Gain  Gain=9/2
  Product2 : Product
  Product3 : Product
  Product9 : Product
  Sum3 : Sum  Inputs=-|+
  M_Mi : Outport
  wires:
  Factor/1 -> Product9/1  "M_Mi"
  polepairs/1 -> Product9/2
  Product9/1 -> M_Mi/1  "M_Mi"
  I_q/1 -> Product3/2
  I_d/1 -> Product2/1
  psi_d/1 -> Product3/1
  psi_q/1 -> Product2/2
  Product2/1 -> Sum3/1
  Product3/1 -> Sum3/2
  Sum3/1 -> Factor/1

== system gm_uz_pmsm_model_9ph_21b_all_double_vnl/uz_pmsm_model_9ph_vnl/dq_model_9ph/mechanical_system/integrator ==
  in : Inport
  reset : Inport  Port=2
  Delay1 : Delay  DelayLength=1  ExternalReset=Level
      settings: InputPortMap=u0,r5
  Gain : Gain  Gain=ts  OutDataTypeStr=Inherit: Same as input
  Sum3 : Sum  Inputs=|++  OutDataTypeStr=Inherit: Same as first input
  outt : Outport
  wires:
  Sum3/1 -> Delay1/1
  Delay1/1 -> Sum3/2, outt/1
  in/1 -> Gain/1
  Gain/1 -> Sum3/1
  reset/1 -> Delay1/2

== system gm_uz_pmsm_model_9ph_21b_all_double_vnl/uz_pmsm_model_9ph_vnl/dq_model_9ph/pmsm/integrator ==
  in : Inport
  reset : Inport  Port=2
  Delay1 : Delay  DelayLength=1  ExternalReset=Level
      settings: InputPortMap=u0,r5
  Gain : Gain  Gain=ts  OutDataTypeStr=Inherit: Same as input
  Sum3 : Sum  Inputs=|++  OutDataTypeStr=Inherit: Same as first input
  outt : Outport
  wires:
  Sum3/1 -> Delay1/1
  Delay1/1 -> Sum3/2, outt/1
  in/1 -> Gain/1
  Gain/1 -> Sum3/1
  reset/1 -> Delay1/2

== system gm_uz_pmsm_model_9ph_21b_all_double_vnl/uz_pmsm_model_9ph_vnl/dq_model_9ph/pmsm/integrator1 ==
  in : Inport
  reset : Inport  Port=2
  Delay1 : Delay  DelayLength=1  ExternalReset=Level
      settings: InputPortMap=u0,r5
  Gain : Gain  Gain=ts  OutDataTypeStr=Inherit: Same as input
  Sum3 : Sum  Inputs=|++  OutDataTypeStr=Inherit: Same as first input
  outt : Outport
  wires:
  Sum3/1 -> Delay1/1
  Delay1/1 -> Sum3/2, outt/1
  in/1 -> Gain/1
  Gain/1 -> Sum3/1
  reset/1 -> Delay1/2

== system gm_uz_pmsm_model_9ph_21b_all_double_vnl/uz_pmsm_model_9ph_vnl/dq_model_9ph/pmsm/integrator2 ==
  in : Inport
  reset : Inport  Port=2
  Delay1 : Delay  DelayLength=1  ExternalReset=Level
      settings: InputPortMap=u0,r5
  Gain : Gain  Gain=ts  OutDataTypeStr=Inherit: Same as input
  Sum3 : Sum  Inputs=|++  OutDataTypeStr=Inherit: Same as first input
  outt : Outport
  wires:
  Sum3/1 -> Delay1/1
  Delay1/1 -> Sum3/2, outt/1
  in/1 -> Gain/1
  Gain/1 -> Sum3/1
  reset/1 -> Delay1/2

== system gm_uz_pmsm_model_9ph_21b_all_double_vnl/uz_pmsm_model_9ph_vnl/dq_model_9ph/pmsm/integrator3 ==
  in : Inport
  reset : Inport  Port=2
  Delay1 : Delay  DelayLength=1  ExternalReset=Level
      settings: InputPortMap=u0,r5
  Gain : Gain  Gain=ts  OutDataTypeStr=Inherit: Same as input
  Sum3 : Sum  Inputs=|++  OutDataTypeStr=Inherit: Same as first input
  outt : Outport
  wires:
  Sum3/1 -> Delay1/1
  Delay1/1 -> Sum3/2, outt/1
  in/1 -> Gain/1
  Gain/1 -> Sum3/1
  reset/1 -> Delay1/2

== system gm_uz_pmsm_model_9ph_21b_all_double_vnl/uz_pmsm_model_9ph_vnl/dq_model_9ph/pmsm/integrator4 ==
  in : Inport
  reset : Inport  Port=2
  Delay1 : Delay  DelayLength=1  ExternalReset=Level
      settings: InputPortMap=u0,r5
  Gain : Gain  Gain=ts  OutDataTypeStr=Inherit: Same as input
  Sum3 : Sum  Inputs=|++  OutDataTypeStr=Inherit: Same as first input
  outt : Outport
  wires:
  Sum3/1 -> Delay1/1
  Delay1/1 -> Sum3/2, outt/1
  in/1 -> Gain/1
  Gain/1 -> Sum3/1
  reset/1 -> Delay1/2

== system gm_uz_pmsm_model_9ph_21b_all_double_vnl/uz_pmsm_model_9ph_vnl/dq_model_9ph/pmsm/integrator5 ==
  in : Inport
  reset : Inport  Port=2
  Delay1 : Delay  DelayLength=1  ExternalReset=Level
      settings: InputPortMap=u0,r5
  Gain : Gain  Gain=ts  OutDataTypeStr=Inherit: Same as input
  Sum3 : Sum  Inputs=|++  OutDataTypeStr=Inherit: Same as first input
  outt : Outport
  wires:
  Sum3/1 -> Delay1/1
  Delay1/1 -> Sum3/2, outt/1
  in/1 -> Gain/1
  Gain/1 -> Sum3/1
  reset/1 -> Delay1/2

== system gm_uz_pmsm_model_9ph_21b_all_double_vnl/uz_pmsm_model_9ph_vnl/dq_model_9ph/pmsm/integrator6 ==
  in : Inport
  reset : Inport  Port=2
  Delay1 : Delay  DelayLength=1  ExternalReset=Level
      settings: InputPortMap=u0,r5
  Gain : Gain  Gain=ts  OutDataTypeStr=Inherit: Same as input
  Sum3 : Sum  Inputs=|++  OutDataTypeStr=Inherit: Same as first input
  outt : Outport
  wires:
  Sum3/1 -> Delay1/1
  Delay1/1 -> Sum3/2, outt/1
  in/1 -> Gain/1
  Gain/1 -> Sum3/1
  reset/1 -> Delay1/2

== system gm_uz_pmsm_model_9ph_21b_all_double_vnl/uz_pmsm_model_9ph_vnl/dq_model_9ph/pmsm/integrator7 ==
  in : Inport
  reset : Inport  Port=2
  Delay1 : Delay  DelayLength=1  ExternalReset=Level
      settings: InputPortMap=u0,r5
  Gain : Gain  Gain=ts  OutDataTypeStr=Inherit: Same as input
  Sum3 : Sum  Inputs=|++  OutDataTypeStr=Inherit: Same as first input
  outt : Outport
  wires:
  Sum3/1 -> Delay1/1
  Delay1/1 -> Sum3/2, outt/1
  in/1 -> Gain/1
  Gain/1 -> Sum3/1
  reset/1 -> Delay1/2

== system gm_uz_pmsm_model_9ph_21b_all_double_vnl/uz_pmsm_model_9ph_vnl/dq_model_9ph/pmsm/integrator8 ==
  in : Inport
  reset : Inport  Port=2
  Delay1 : Delay  DelayLength=1  ExternalReset=Level
      settings: InputPortMap=u0,r5
  Gain : Gain  Gain=ts  OutDataTypeStr=Inherit: Same as input
  Sum3 : Sum  Inputs=|++  OutDataTypeStr=Inherit: Same as first input
  outt : Outport
  wires:
  Sum3/1 -> Delay1/1
  Delay1/1 -> Sum3/2, outt/1
  in/1 -> Gain/1
  Gain/1 -> Sum3/1
  reset/1 -> Delay1/2

== matlab function gm_uz_pmsm_model_9ph_21b_all_double_vnl/Compare/Assert_outputs/RelErrCheck/RelativeErrorCheck  ==
  data: P input; y output; R input; ToleranceValue parameter double
% Check if the relative error of R with respect to P is below
% ToleranceValue
% P, R are floating-point
function y = relErrCheck(P,R, ToleranceValue)
    tol = ToleranceValue;
    sz = numel(P);
    assert(sz == numel(R), 'Inputs P and R have different sizes.');
    y = false(1, sz);

    for ii=1:sz
        if (isnan(P(ii)) || isnan(R(ii)))
            if (isnan(P(ii)) && isnan(R(ii)))
                y(ii) = true;
            end
        elseif (isinf(P(ii)) || isinf(R(ii)))
            y(ii) = (P(ii) == R(ii));
        elseif (P(ii) == 0)
            y(ii) = (R(ii) == 0);
        else
            absdiff = abs(P(ii) - R(ii));
            relerr = absdiff/abs(P(ii));
            y(ii) = (relerr <= tol);
        end
    end
end

== matlab function gm_uz_pmsm_model_9ph_21b_all_double_vnl/Compare/Assert_i_abc_ps/RelErrCheck/RelativeErrorCheck  ==
  data: P input; y output; R input; ToleranceValue parameter double
% Check if the relative error of R with respect to P is below
% ToleranceValue
% P, R are floating-point
function y = relErrCheck(P,R, ToleranceValue)
    tol = ToleranceValue;
    sz = numel(P);
    assert(sz == numel(R), 'Inputs P and R have different sizes.');
    y = false(1, sz);

    for ii=1:sz
        if (isnan(P(ii)) || isnan(R(ii)))
            if (isnan(P(ii)) && isnan(R(ii)))
                y(ii) = true;
            end
        elseif (isinf(P(ii)) || isinf(R(ii)))
            y(ii) = (P(ii) == R(ii));
        elseif (P(ii) == 0)
            y(ii) = (R(ii) == 0);
        else
            absdiff = abs(P(ii) - R(ii));
            relerr = absdiff/abs(P(ii));
            y(ii) = (relerr <= tol);
        end
    end
end
